simulink model "enc_eml"  (R2014a)
settings: Solver=FixedStepDiscrete  SolverMode=SingleTasking  StartTime=0.0  StopTime=10.0  RelTol=1e-3
settings Model: ExtModeTrigDuration=2  Creator=gcampa  LastModifiedBy=gcampa
settings OptimizationCC: OptimizeModelRefInitCode=on  LifeSpan=1
settings DebuggingCC: UnderspecifiedInitializationDetection=Classic  SolverPrmCheckMsg=none  FrameProcessingCompatibilityMsg=error  StateNameClashWarn=warning
settings HardwareCC: ProdBitPerInt=16  ProdBitPerPointer=8  ProdIntDivRoundTo=Zero  ProdEndianess=LittleEndian  ProdWordSize=8  ProdHWDeviceType=Atmel->AVR
settings RTWCC: SystemTargetFile=realtime.tlc  GenerateMakefile=off  TemplateMakefile=realtime.tmf  Description=Run on Target Hardware  RTWVerbose=off  ProcessScript=realtime_make_rtw_hook  CustomSource=..\src\encoder_arduino.cpp
settings STFCustomTargetCC: TargetLibSuffix=.a  GenerateSampleERTMain=on  ConcurrentExecutionCompliant=off  GeneratePreprocessorConditionals=Use local settings  ERTCustomFileBanners=on  SupportNonInlinedSFcns=off  SupportVariableSizeSignals=on  MATLABClassNameForMDSCustomization=Simulink.SoftwareTarget.ERTCustomization  GRTInterface=off  SystemTargetFile=realtime.tlc
settings ERTTargetCC: CombineOutputUpdateFcns=off  SupportContinuousTime=on  SupportVariableSizeSignals=on  ExtModeTransport=3  ExtModeMexFile=ext_serial_win32_comm  ExtModeMexArgs=0 1 9600  ERTSrcFileBannerTemplate=realtime_code_template.cgt  ERTHdrFileBannerTemplate=realtime_code_template.cgt  ERTDataSrcFileTemplate=realtime_code_template.cgt  ERTDataHdrFileTemplate=realtime_code_template.cgt  ERTCustomFileTemplate=realtime_file_process.tlc

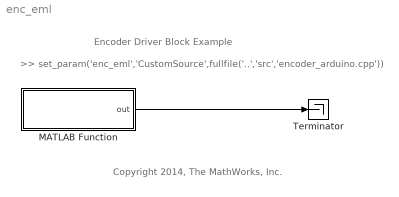
== system enc_eml ==
  note: Encoder Driver Block Example
  note: Copyright 2014, The MathWorks, Inc.
  note: >> set_param('enc_eml','CustomSource',fullfile('..','src','encoder_arduino.cpp'))
  MATLAB Function : MATLAB Function  TreatAsAtomicUnit=on  mask(Encoder Read){enc=0, pinA=2, pinB=3, T=0.05}
      mask prompts: enc "Encoder Number (0, 1 or 2)"; pinA "Pin A"; pinB "Pin B"; T "Sample TIme"
      mask help:
      | At initialization time, this block attaches interrupt service routines (written in eml_enc_src.c) to the two pins (pinA and pinB) to which the encoder is connected (the "common" central pin a.k.a. pinC of the encoder should be connected to ground). After that, when the encoder rotates the interrupts service routines update the encoder position. The encoder position is then set as output of the block every time the block is executed.
      |
      | The first parameter is the encoder identifier, must be either 0, 1 or 2. PinA and PinB are the pins to which the encoder is attached. The allowed pins are 2 and 3 on the Uno board and 2,3,18,19,20,21 on the Mega board. The last parameter is the Sample Time.
      |
      | Note that if this block gets copied to a new model, then the file "encoder_arduino.cpp" must be added to the CustomSource field of the new model using the "set_param" instruction. See the guide for more info.
  Terminator : Terminator
  wires:
  MATLAB Function/1(out) -> Terminator/1

== matlab function enc_eml/MATLAB Function ==
  settings: updateMethod=DISCRETE  sampleTime=T
  data: enc parameter int32; out output; pinA parameter int32; pinB parameter uint8
function out = encoderRead(enc,pinA,pinB)
%#codegen

persistent initflag;
out=0;

if strcmp(coder.target, 'rtw'),
    
    if isempty(initflag),
        % Initialize step
        coder.ceval('enc_init',int16(enc),int16(pinA),int16(pinB));
        initflag = 1;
    else
        % output Step
        out=coder.ceval('enc_output',int16(enc));
    end
    
end
